simulink model "electromagnet_d"  (R2024a)
settings: Solver=VariableStepAuto  StartTime=0.0  StopTime=te  MaxStep=te/100  RelTol=1e-3
values from neighbouring files (symbols this model uses):
  m = 3    [sim21_solution.m]
  x0 = [0 0]    [sim21_solution.m]
undefined symbols (not defined in the file or in its folder): Amplitude, g, Period, PulseWidth
settings Model: Creator=ocean  LastModifiedBy=ocean

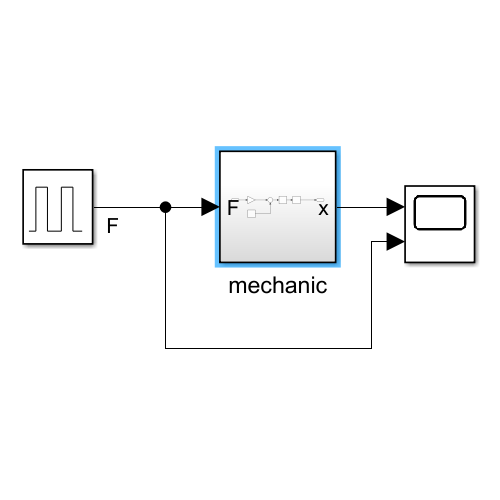
[thumbnail: Simulink's stored preview of the top-level diagram]
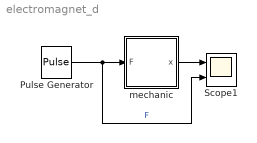
== system electromagnet_d ==
  Pulse Generator : DiscretePulseGenerator  PulseType=Time based  Amplitude=Amplitude  Period=Period  PulseWidth=PulseWidth
  Scope1 : Scope  NumInputPorts=2
  mechanic : Subsystem
  wires:
  Pulse Generator/1 -> Scope1/2, mechanic/1(F)  "F"
  mechanic/1(x) -> Scope1/1

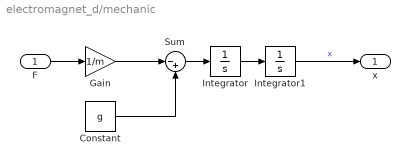
== system electromagnet_d/mechanic ==
  F : Inport
  Constant : Constant  Value=g
  Gain : Gain  Gain=1/m
  Integrator : Integrator
  Integrator1 : Integrator  InitialCondition=x0
  Sum : Sum  Inputs=|-+
  x : Outport
  wires:
  F/1 -> Gain/1
  Constant/1 -> Sum/2
  Gain/1 -> Sum/1
  Integrator/1 -> Integrator1/1
  Integrator1/1 -> x/1  "x"
  Sum/1 -> Integrator/1
